simulink model "construction_robots"  (Simulink 9.2)
settings: Solver=VariableStepAuto  StartTime=0.0  StopTime=30  MaxStep=1e-4  RelTol=1e-5
settings Model: Creator=jinwooro  LastModifiedBy=jinwooro  PauseTimes=19
settings SolverCC: ZeroCrossAlgorithm=Adaptive
settings DataIOCC: LimitDataPoints=off  SaveFormat=Dataset  SignalLoggingSaveFormat=Dataset
settings OptimizationCC: LifeSpan=auto
settings DebuggingCC: UnderspecifiedInitializationDetection=Simplified  MergeDetectMultiDrivingBlocksExec=error  FcnCallInpInsideContextMsg=error  StateNameClashWarn=none  SFUnexpectedBacktrackingDiag=error  SFNoUnconditionalDefaultTransitionDiag=error  SFExecutionAtInitializationDiag=warning
settings HardwareCC: ProdBitPerPointer=64  ProdBitPerSizeT=64  ProdBitPerPtrDiffT=64  ProdLargestAtomicFloat=Float  ProdIntDivRoundTo=Zero  ProdEndianess=LittleEndian  ProdWordSize=64  ProdHWDeviceType=Intel->x86-64 (Windows64)
settings ModelReferenceCC: PropagateSignalLabelsOutOfModel=on
settings SFSimCC: SimUseLocalCustomCode=on
settings RTWCC: RTWUseLocalCustomCode=on
settings CodeAppCC: StateflowObjectComments=off
settings GRTTargetCC: TargetLangStandard=C99 (ISO)  GeneratePreprocessorConditionals=Use local settings  CombineOutputUpdateFcns=on  GRTInterface=off
settings ConfigComp: CovMetricSettings=dwe  CovHtmlReporting=off  CovSaveCumulativeToWorkspaceVar=off  CovSaveSingleToWorkspaceVar=off  CovExternalEMLEnable=on

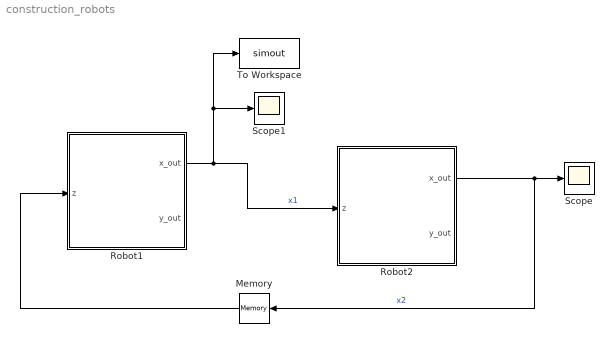
== system construction_robots ==
  Memory : Memory
  Robot1 : Stateflow chart  TreatAsAtomicUnit=on
  Robot2 : Stateflow chart  TreatAsAtomicUnit=on
  Scope : Scope
  Scope1 : Scope
  To Workspace : ToWorkspace  VariableName=simout  SaveFormat=Timeseries  SampleTime=-1
  wires:
  Robot2/1(x_out) -> Scope/1, Memory/1  "x2"
  Robot1/1(x_out) -> To Workspace/1, Scope1/1, Robot2/1(z)  "x1"
  Memory/1 -> Robot1/1(z)

== stateflow chart Robot2 ==
  settings: updateMethod=CONTINUOUS
  state Approach
    du:
    x_dot = 0.5 * (24 - x);
    y_dot = 0;
    x_out = x;
    y_out = y;
  state Wait
    du:
    x_dot = 0;
    x_out = x;
    y_dot = 0;
    y_out = y;
  state Transport
    du:
    x_dot = 0;
    x_out = x;
    y_dot = 1;
    y_out = y;
  (default) -> Approach : {
      | x = 30;
      | y = 0;
      | }
  Approach -> Wait : [abs(25 - x) <= 0.001]{x=25;}
  Wait -> Transport : [abs(x-z) <= 5]
  data: x local double; x_out output double; z input double; y local double; y_out output double
  data x settings: updateMethod=SF_CONTINUOUS_TIME_DATA
  data y settings: updateMethod=SF_CONTINUOUS_TIME_DATA

== stateflow chart Robot1 ==
  settings: updateMethod=CONTINUOUS
  state Approach
    du:
    x_dot = 0.5 * (21 - x);
    y_dot = 0;
    x_out = x;
    y_out = y;
  state Wait
    du:
    x_dot = 0;
    x_out = x;
    y_dot = 0;
    y_out = y;
  state Transport
    du:
    x_dot = 0;
    x_out = x;
    y_dot = 1;
    y_out = y;
  (default) -> Approach : {
      | x = 0;
      | y = 0;
      | }
  Approach -> Wait : [abs(20-x) <= 0.001]{x=20;}
  Wait -> Transport : [abs(x-z) <= 5]
  data: x local double; x_out output double; z input double; y local double; y_out output double
  data x settings: updateMethod=SF_CONTINUOUS_TIME_DATA
  data y settings: updateMethod=SF_CONTINUOUS_TIME_DATA
